simulink model "NORMAL_forces"  (R2015a)
settings: Solver=ode45  StartTime=0.0  StopTime=10.0  RelTol=1e-3
undefined symbols (not defined in the file): h, l, l_f, l_r, l_w, m
settings Model: Creator=BML  LastModifiedBy=BML

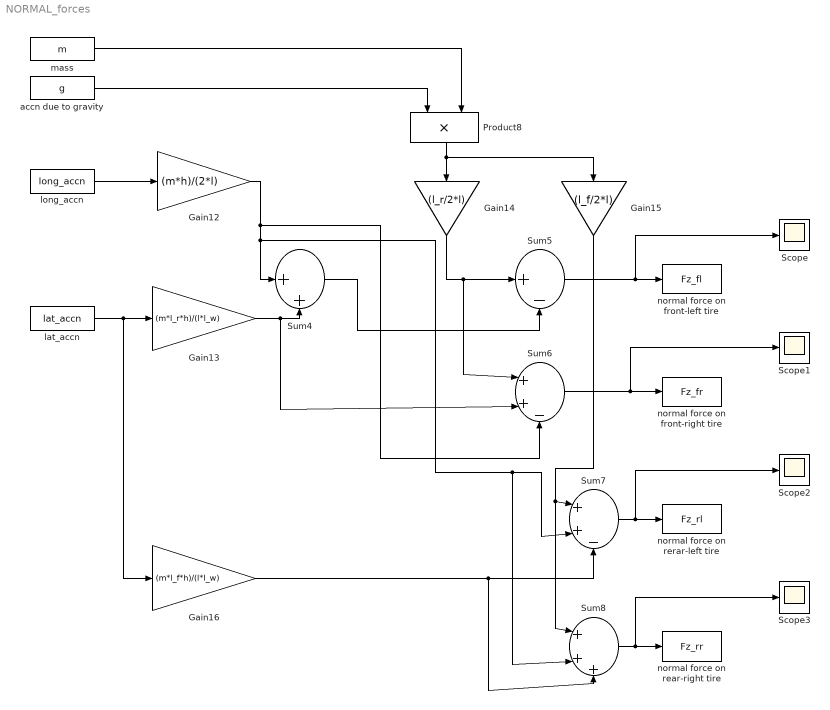
== system NORMAL_forces ==
  Gain12 : Gain  Gain=(m*h)/(2*l)
  Gain13 : Gain  Gain=(m*l_r*h)/(l*l_w)
  Gain14 : Gain  Gain=(l_r/2*l)
  Gain15 : Gain  Gain=(l_f/2*l)
  Gain16 : Gain  Gain=(m*l_f*h)/(l*l_w)
  Product8 : Product
  Scope{,1..3} (4 alike) : Scope
      Scope2 settings: SaveName=ScopeData2
      Scope3 settings: SaveName=ScopeData3
  Sum4 : Sum  Inputs=|++
  Sum5 : Sum  Inputs=|+-
  Sum6 : Sum  Inputs=|++-
  Sum7 : Sum  Inputs=|++-
  Sum8 : Sum  Inputs=|+++
  accn due to gravity : FromWorkspace  VariableName=g  SampleTime=0
  lat_accn : FromWorkspace  VariableName=lat_accn  SampleTime=0
  long_accn : FromWorkspace  VariableName=long_accn  SampleTime=0
  mass : FromWorkspace  VariableName=m  SampleTime=0
  normal force on front-left tire : ToWorkspace  VariableName=Fz_fl  SaveFormat=Timeseries  SampleTime=-1
  normal force on front-right tire : ToWorkspace  VariableName=Fz_fr  SaveFormat=Timeseries  SampleTime=-1
  normal force on rear-right tire : ToWorkspace  VariableName=Fz_rr  SaveFormat=Timeseries  SampleTime=-1
  normal force on rerar-left tire : ToWorkspace  VariableName=Fz_rl  SaveFormat=Timeseries  SampleTime=-1
  wires:
  accn due to gravity/1 -> Product8/1
  Product8/1 -> Gain15/1, Gain14/1
  mass/1 -> Product8/2
  long_accn/1 -> Gain12/1
  lat_accn/1 -> Gain16/1, Gain13/1
  Gain13/1 -> Sum6/2, Sum4/2
  Gain12/1 -> Sum4/1, Sum8/2, Sum7/2, Sum6/3
  Gain14/1 -> Sum5/1, Sum6/1
  Sum4/1 -> Sum5/2
  Sum5/1 -> Scope/1, normal force on front-left tire/1
  Gain15/1 -> Sum8/1, Sum7/1
  Gain16/1 -> Sum8/3, Sum7/3
  Sum6/1 -> normal force on front-right tire/1, Scope1/1
  Sum7/1 -> Scope2/1, normal force on rerar-left tire/1
  Sum8/1 -> Scope3/1, normal force on rear-right tire/1
